simulink model "mixer_old"  (R2024b)
settings: Solver=FixedStepAuto  StartTime=0.0  StopTime=10.0  RelTol=1e-3
undefined symbols (not defined in the file or in its folder): MC_AIRMODE, MOT_SLEW_MAX, THR_MDL_FAC
libraries: simulink x58
(part 2 of 3)

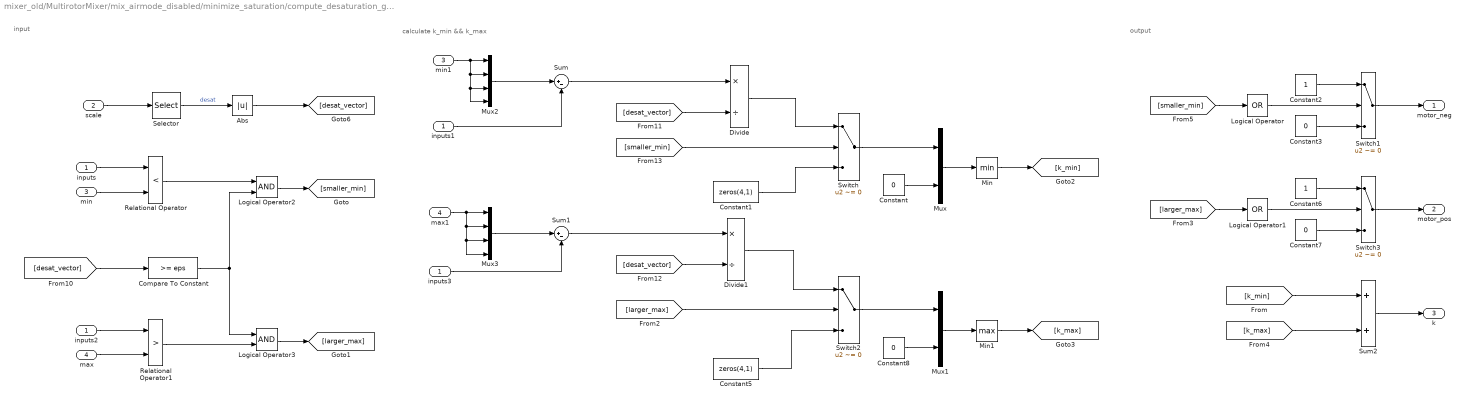
== system mixer_old/MultirotorMixer/mix_airmode_disabled/minimize_saturation/compute_desaturation_gain ==
  note: input
  note: output
  note: calculate k_min && k_max
  inputs : Inport
  scale : Inport  Port=2
  min : Inport  Port=3
  max : Inport  Port=4
  Abs : Abs  SaturateOnIntegerOverflow=off
  Compare To Constant : simulink/Logic and Bit Operations/Compare To Constant  relop=>=  const=eps  OutDataTypeStr=boolean
      settings: AttributesFormatString=%<relop>%<const>
  Constant{,3,7..8} (4 alike) : Constant  Value=0  OutDataTypeStr=single
  Constant1 : Constant  Value=zeros(4,1)  OutDataTypeStr=single
  Constant2 : Constant  OutDataTypeStr=single
  Constant5 : Constant  Value=zeros(4,1)  OutDataTypeStr=single
  Constant6 : Constant  OutDataTypeStr=single
  Divide : Product  Inputs=*/
  Divide1 : Product  Inputs=*/
  Logical Operator : Logic  Operator=OR  Inputs=1  AllPortsSameDT=off  OutDataTypeStr=boolean
  Logical Operator1 : Logic  Operator=OR  Inputs=1  AllPortsSameDT=off  OutDataTypeStr=boolean
  Logical Operator2 : Logic  AllPortsSameDT=off  OutDataTypeStr=boolean
  Logical Operator3 : Logic  AllPortsSameDT=off  OutDataTypeStr=boolean
  Min : MinMax
  Min1 : MinMax  Function=max
  Mux : Mux  Inputs=2
  Mux1 : Mux  Inputs=2
  Mux2 : Mux
  Mux3 : Mux
  Relational Operator : RelationalOperator  Operator=<  OutDataTypeStr=boolean  RndMeth=Simplest  InputSameDT=off
  Relational Operator1 : RelationalOperator  Operator=>  OutDataTypeStr=boolean  RndMeth=Simplest  InputSameDT=off
  Selector : Selector  NumberOfDimensions=2  InputPortWidth=3  IndexOptions=Select all,Index vector (dialog)  Indices=[1 3],4  OutputSizes=1,1
  Sum : Sum  Inputs=|+-
  Sum1 : Sum  Inputs=|+-
  Sum2 : Sum
  Switch{,1..3} (4 alike) : Switch  Criteria=u2 ~= 0  SaturateOnIntegerOverflow=off  InputSameDT=off
  inputs1 : InportShadow
  inputs2 : InportShadow
  inputs3 : InportShadow
  max1 : InportShadow  Port=4
  min1 : InportShadow  Port=3
  motor_neg : Outport
  motor_pos : Outport  Port=2
  k : Outport  Port=3
  wires:
  inputs/1 -> Relational Operator/1
  Mux2/1 -> Sum/1
  inputs1/1 -> Sum/2
  Sum/1 -> Divide/1
  [desat_vector] -> Divide/2
  Divide/1 -> Switch/1
  Constant1/1 -> Switch/3
  Logical Operator/1 -> Switch1/2
  Constant2/1 -> Switch1/1
  Constant3/1 -> Switch1/3
  Switch1/1 -> motor_neg/1
  inputs2/1 -> Relational Operator1/1
  [larger_max] -> Switch2/2
  Mux3/1 -> Sum1/1
  inputs3/1 -> Sum1/2
  [desat_vector] -> Divide1/2
  Sum1/1 -> Divide1/1
  Divide1/1 -> Switch2/1
  Constant5/1 -> Switch2/3
  Constant7/1 -> Switch3/3
  Constant6/1 -> Switch3/1
  Logical Operator1/1 -> Switch3/2
  Switch3/1 -> motor_pos/1
  Relational Operator/1 -> Logical Operator2/1
  [smaller_min] -> Logical Operator/1
  Relational Operator1/1 -> Logical Operator3/2
  [larger_max] -> Logical Operator1/1
  Sum2/1 -> k/1
  Compare To Constant/1 -> Logical Operator2/2, Logical Operator3/1
  Logical Operator2/1 -> [smaller_min]
  Logical Operator3/1 -> [larger_max]
  min/1 -> Relational Operator/2
  max/1 -> Relational Operator1/2
  min1/1 -> Mux2/4, Mux2/3, Mux2/2, Mux2/1
  max1/1 -> Mux3/2, Mux3/3, Mux3/4, Mux3/1
  scale/1 -> Selector/1
  Selector/1 -> Abs/1  "desat"
  Abs/1 -> [desat_vector]
  [desat_vector] -> Compare To Constant/1
  [smaller_min] -> Switch/2
  Min/1 -> [k_min]
  Min1/1 -> [k_max]
  Switch/1 -> Mux/1
  Constant/1 -> Mux/2
  Mux/1 -> Min/1
  Mux1/1 -> Min1/1
  Constant8/1 -> Mux1/2
  Switch2/1 -> Mux1/1
  [k_min] -> Sum2/1
  [k_max] -> Sum2/2

== system mixer_old/MultirotorMixer/mix_airmode_disabled/minimize_saturation1/If Action Subsystem ==
  motor_neg : Inport
  motor_pos : Inport  Port=2
  outputs : Inport  Port=3
  Action Port : ActionPort  ActionPortLabel=if(u1)
  Bus Creator : BusCreator  Inputs=3
  out : Outport
  wires:
  Bus Creator/1 -> out/1
  outputs/1 -> Bus Creator/3  "outputs"
  motor_neg/1 -> Bus Creator/1  "motor_neg"
  motor_pos/1 -> Bus Creator/2  "motor_pos"

== system mixer_old/MultirotorMixer/mix_airmode_disabled/minimize_saturation1/Subsystem ==
  k1 : Inport
  scale : Inport  Port=2
  inputs : Inport  Port=3
  Action Port : ActionPort  ActionPortLabel=else
  Bus Creator1 : BusCreator  Inputs=3
  Constant1 : Constant  Value=0  OutDataTypeStr=single
  Constant2 : Constant  OutDataTypeStr=single
  Gain : Gain  Gain=0.5
  Product : Product
  Product1 : Product
  Selector : Selector  NumberOfDimensions=2  InputPortWidth=3  IndexOptions=Select all,Index vector (dialog)  Indices=[1 3],4  OutputSizes=1,1
  Selector1 : Selector  NumberOfDimensions=2  InputPortWidth=3  IndexOptions=Select all,Index vector (dialog)  Indices=[1 3],4  OutputSizes=1,1
  Sum : Sum  Inputs=++|
  Sum1 : Sum  Inputs=|++
  compute_desaturation_gain : Subsystem
  scale1 : InportShadow  Port=2
  scale2 : InportShadow  Port=2
  out : Outport
  wires:
  Selector1/1 -> Product1/2  "desat"
  scale2/1 -> Selector1/1
  scale1/1 -> compute_desaturation_gain/2(scale)
  inputs/1 -> Sum/1
  Product/1 -> Sum/2
  Selector/1 -> Product/2  "desat"
  Constant2/1 -> compute_desaturation_gain/4(max)
  Constant1/1 -> compute_desaturation_gain/3(min)
  k1/1 -> Product/1
  Gain/1 -> Product1/1  "k2"
  Bus Creator1/1 -> out/1
  compute_desaturation_gain/1(motor_neg) -> Bus Creator1/1  "motor_neg"
  Product1/1 -> Sum1/1
  compute_desaturation_gain/3(k) -> Gain/1
  Sum1/1 -> Bus Creator1/3  "outputs"
  compute_desaturation_gain/2(motor_pos) -> Bus Creator1/2  "motor_pos"
  scale/1 -> Selector/1
  Sum/1 -> Sum1/2, compute_desaturation_gain/1(inputs)

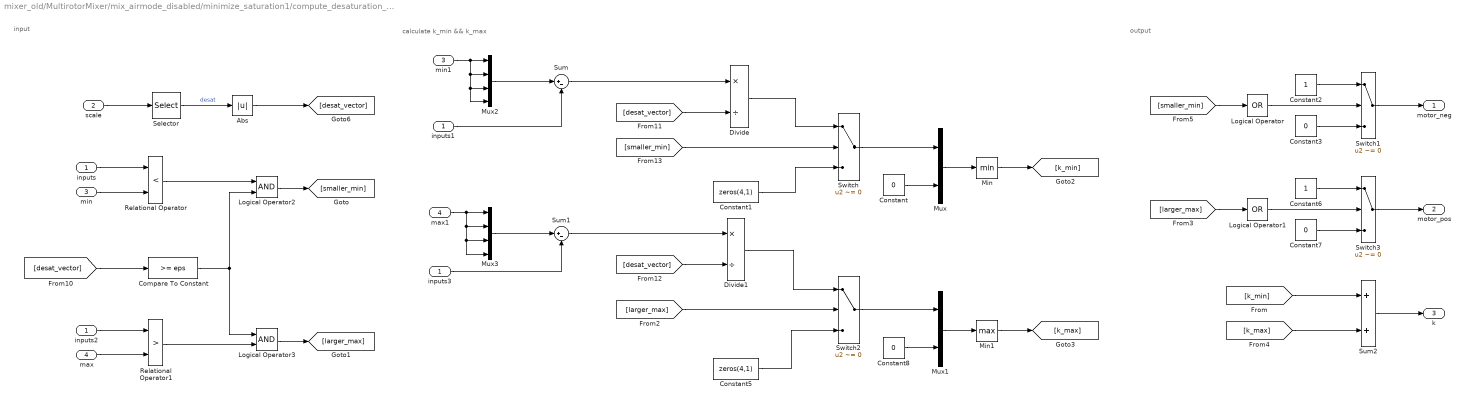
== system mixer_old/MultirotorMixer/mix_airmode_disabled/minimize_saturation1/compute_desaturation_gain ==
  note: calculate k_min && k_max
  note: output
  note: input
  inputs : Inport
  scale : Inport  Port=2
  min : Inport  Port=3
  max : Inport  Port=4
  Abs : Abs  SaturateOnIntegerOverflow=off
  Compare To Constant : simulink/Logic and Bit Operations/Compare To Constant  relop=>=  const=eps  OutDataTypeStr=boolean
      settings: AttributesFormatString=%<relop>%<const>
  Constant{,3,7..8} (4 alike) : Constant  Value=0  OutDataTypeStr=single
  Constant1 : Constant  Value=zeros(4,1)  OutDataTypeStr=single
  Constant2 : Constant  OutDataTypeStr=single
  Constant5 : Constant  Value=zeros(4,1)  OutDataTypeStr=single
  Constant6 : Constant  OutDataTypeStr=single
  Divide : Product  Inputs=*/
  Divide1 : Product  Inputs=*/
  Logical Operator : Logic  Operator=OR  Inputs=1  AllPortsSameDT=off  OutDataTypeStr=boolean
  Logical Operator1 : Logic  Operator=OR  Inputs=1  AllPortsSameDT=off  OutDataTypeStr=boolean
  Logical Operator2 : Logic  AllPortsSameDT=off  OutDataTypeStr=boolean
  Logical Operator3 : Logic  AllPortsSameDT=off  OutDataTypeStr=boolean
  Min : MinMax
  Min1 : MinMax  Function=max
  Mux : Mux  Inputs=2
  Mux1 : Mux  Inputs=2
  Mux2 : Mux
  Mux3 : Mux
  Relational Operator : RelationalOperator  Operator=<  OutDataTypeStr=boolean  RndMeth=Simplest  InputSameDT=off
  Relational Operator1 : RelationalOperator  Operator=>  OutDataTypeStr=boolean  RndMeth=Simplest  InputSameDT=off
  Selector : Selector  NumberOfDimensions=2  InputPortWidth=3  IndexOptions=Select all,Index vector (dialog)  Indices=[1 3],4  OutputSizes=1,1
  Sum : Sum  Inputs=|+-
  Sum1 : Sum  Inputs=|+-
  Sum2 : Sum
  Switch{,1..3} (4 alike) : Switch  Criteria=u2 ~= 0  SaturateOnIntegerOverflow=off  InputSameDT=off
  inputs1 : InportShadow
  inputs2 : InportShadow
  inputs3 : InportShadow
  max1 : InportShadow  Port=4
  min1 : InportShadow  Port=3
  motor_neg : Outport
  motor_pos : Outport  Port=2
  k : Outport  Port=3
  wires:
  [k_max] -> Sum2/2
  [k_min] -> Sum2/1
  Switch2/1 -> Mux1/1
  Constant8/1 -> Mux1/2
  Mux1/1 -> Min1/1
  Mux/1 -> Min/1
  Constant/1 -> Mux/2
  Switch/1 -> Mux/1
  Min1/1 -> [k_max]
  Min/1 -> [k_min]
  [smaller_min] -> Switch/2
  [desat_vector] -> Compare To Constant/1
  Abs/1 -> [desat_vector]
  Selector/1 -> Abs/1  "desat"
  scale/1 -> Selector/1
  max1/1 -> Mux3/1, Mux3/4, Mux3/3, Mux3/2
  min1/1 -> Mux2/1, Mux2/2, Mux2/3, Mux2/4
  max/1 -> Relational Operator1/2
  min/1 -> Relational Operator/2
  Logical Operator3/1 -> [larger_max]
  Logical Operator2/1 -> [smaller_min]
  Compare To Constant/1 -> Logical Operator3/1, Logical Operator2/2
  Sum2/1 -> k/1
  [larger_max] -> Logical Operator1/1
  Relational Operator1/1 -> Logical Operator3/2
  [smaller_min] -> Logical Operator/1
  Relational Operator/1 -> Logical Operator2/1
  Switch3/1 -> motor_pos/1
  Logical Operator1/1 -> Switch3/2
  Constant6/1 -> Switch3/1
  Constant7/1 -> Switch3/3
  Constant5/1 -> Switch2/3
  Divide1/1 -> Switch2/1
  Sum1/1 -> Divide1/1
  [desat_vector] -> Divide1/2
  inputs3/1 -> Sum1/2
  Mux3/1 -> Sum1/1
  [larger_max] -> Switch2/2
  inputs2/1 -> Relational Operator1/1
  Switch1/1 -> motor_neg/1
  Constant3/1 -> Switch1/3
  Constant2/1 -> Switch1/1
  Logical Operator/1 -> Switch1/2
  Constant1/1 -> Switch/3
  Divide/1 -> Switch/1
  [desat_vector] -> Divide/2
  Sum/1 -> Divide/1
  inputs1/1 -> Sum/2
  Mux2/1 -> Sum/1
  inputs/1 -> Relational Operator/1

== system mixer_old/MultirotorMixer/mix_airmode_disabled/minimize_saturation2/If Action Subsystem ==
  motor_neg : Inport
  motor_pos : Inport  Port=2
  outputs : Inport  Port=3
  Action Port : ActionPort  ActionPortLabel=if(u1)
  Bus Creator : BusCreator  Inputs=3
  out : Outport
  wires:
  motor_pos/1 -> Bus Creator/2  "motor_pos"
  motor_neg/1 -> Bus Creator/1  "motor_neg"
  outputs/1 -> Bus Creator/3  "outputs"
  Bus Creator/1 -> out/1

== system mixer_old/MultirotorMixer/mix_airmode_disabled/minimize_saturation2/Subsystem ==
  k1 : Inport
  scale : Inport  Port=2
  inputs : Inport  Port=3
  Action Port : ActionPort  ActionPortLabel=else
  Bus Creator1 : BusCreator  Inputs=3
  Constant1 : Constant  Value=0  OutDataTypeStr=single
  Constant2 : Constant  OutDataTypeStr=single
  Gain : Gain  Gain=0.5
  Product : Product
  Product1 : Product
  Selector : Selector  NumberOfDimensions=2  InputPortWidth=3  IndexOptions=Select all,Index vector (dialog)  Indices=[1 3],4  OutputSizes=1,1
  Selector1 : Selector  NumberOfDimensions=2  InputPortWidth=3  IndexOptions=Select all,Index vector (dialog)  Indices=[1 3],4  OutputSizes=1,1
  Sum : Sum  Inputs=++|
  Sum1 : Sum  Inputs=|++
  compute_desaturation_gain : Subsystem
  scale1 : InportShadow  Port=2
  scale2 : InportShadow  Port=2
  out : Outport
  wires:
  Sum/1 -> compute_desaturation_gain/1(inputs), Sum1/2
  scale/1 -> Selector/1
  compute_desaturation_gain/2(motor_pos) -> Bus Creator1/2  "motor_pos"
  Sum1/1 -> Bus Creator1/3  "outputs"
  compute_desaturation_gain/3(k) -> Gain/1
  Product1/1 -> Sum1/1
  compute_desaturation_gain/1(motor_neg) -> Bus Creator1/1  "motor_neg"
  Bus Creator1/1 -> out/1
  Gain/1 -> Product1/1  "k2"
  k1/1 -> Product/1
  Constant1/1 -> compute_desaturation_gain/3(min)
  Constant2/1 -> compute_desaturation_gain/4(max)
  Selector/1 -> Product/2  "desat"
  Product/1 -> Sum/2
  inputs/1 -> Sum/1
  scale1/1 -> compute_desaturation_gain/2(scale)
  scale2/1 -> Selector1/1
  Selector1/1 -> Product1/2  "desat"

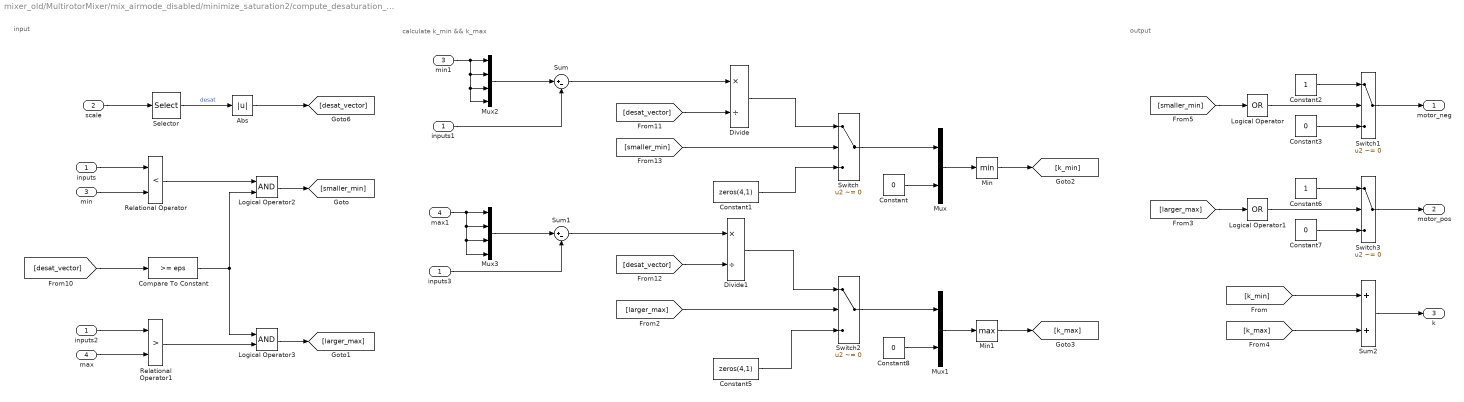
== system mixer_old/MultirotorMixer/mix_airmode_disabled/minimize_saturation2/compute_desaturation_gain ==
  note: input
  note: output
  note: calculate k_min && k_max
  inputs : Inport
  scale : Inport  Port=2
  min : Inport  Port=3
  max : Inport  Port=4
  Abs : Abs  SaturateOnIntegerOverflow=off
  Compare To Constant : simulink/Logic and Bit Operations/Compare To Constant  relop=>=  const=eps  OutDataTypeStr=boolean
      settings: AttributesFormatString=%<relop>%<const>
  Constant{,3,7..8} (4 alike) : Constant  Value=0  OutDataTypeStr=single
  Constant1 : Constant  Value=zeros(4,1)  OutDataTypeStr=single
  Constant2 : Constant  OutDataTypeStr=single
  Constant5 : Constant  Value=zeros(4,1)  OutDataTypeStr=single
  Constant6 : Constant  OutDataTypeStr=single
  Divide : Product  Inputs=*/
  Divide1 : Product  Inputs=*/
  Logical Operator : Logic  Operator=OR  Inputs=1  AllPortsSameDT=off  OutDataTypeStr=boolean
  Logical Operator1 : Logic  Operator=OR  Inputs=1  AllPortsSameDT=off  OutDataTypeStr=boolean
  Logical Operator2 : Logic  AllPortsSameDT=off  OutDataTypeStr=boolean
  Logical Operator3 : Logic  AllPortsSameDT=off  OutDataTypeStr=boolean
  Min : MinMax
  Min1 : MinMax  Function=max
  Mux : Mux  Inputs=2
  Mux1 : Mux  Inputs=2
  Mux2 : Mux
  Mux3 : Mux
  Relational Operator : RelationalOperator  Operator=<  OutDataTypeStr=boolean  RndMeth=Simplest  InputSameDT=off
  Relational Operator1 : RelationalOperator  Operator=>  OutDataTypeStr=boolean  RndMeth=Simplest  InputSameDT=off
  Selector : Selector  NumberOfDimensions=2  InputPortWidth=3  IndexOptions=Select all,Index vector (dialog)  Indices=[1 3],4  OutputSizes=1,1
  Sum : Sum  Inputs=|+-
  Sum1 : Sum  Inputs=|+-
  Sum2 : Sum
  Switch{,1..3} (4 alike) : Switch  Criteria=u2 ~= 0  SaturateOnIntegerOverflow=off  InputSameDT=off
  inputs1 : InportShadow
  inputs2 : InportShadow
  inputs3 : InportShadow
  max1 : InportShadow  Port=4
  min1 : InportShadow  Port=3
  motor_neg : Outport
  motor_pos : Outport  Port=2
  k : Outport  Port=3
  wires:
  inputs/1 -> Relational Operator/1
  Mux2/1 -> Sum/1
  inputs1/1 -> Sum/2
  Sum/1 -> Divide/1
  [desat_vector] -> Divide/2
  Divide/1 -> Switch/1
  Constant1/1 -> Switch/3
  Logical Operator/1 -> Switch1/2
  Constant2/1 -> Switch1/1
  Constant3/1 -> Switch1/3
  Switch1/1 -> motor_neg/1
  inputs2/1 -> Relational Operator1/1
  [larger_max] -> Switch2/2
  Mux3/1 -> Sum1/1
  inputs3/1 -> Sum1/2
  [desat_vector] -> Divide1/2
  Sum1/1 -> Divide1/1
  Divide1/1 -> Switch2/1
  Constant5/1 -> Switch2/3
  Constant7/1 -> Switch3/3
  Constant6/1 -> Switch3/1
  Logical Operator1/1 -> Switch3/2
  Switch3/1 -> motor_pos/1
  Relational Operator/1 -> Logical Operator2/1
  [smaller_min] -> Logical Operator/1
  Relational Operator1/1 -> Logical Operator3/2
  [larger_max] -> Logical Operator1/1
  Sum2/1 -> k/1
  Compare To Constant/1 -> Logical Operator2/2, Logical Operator3/1
  Logical Operator2/1 -> [smaller_min]
  Logical Operator3/1 -> [larger_max]
  min/1 -> Relational Operator/2
  max/1 -> Relational Operator1/2
  min1/1 -> Mux2/4, Mux2/3, Mux2/2, Mux2/1
  max1/1 -> Mux3/2, Mux3/3, Mux3/4, Mux3/1
  scale/1 -> Selector/1
  Selector/1 -> Abs/1  "desat"
  Abs/1 -> [desat_vector]
  [desat_vector] -> Compare To Constant/1
  [smaller_min] -> Switch/2
  Min/1 -> [k_min]
  Min1/1 -> [k_max]
  Switch/1 -> Mux/1
  Constant/1 -> Mux/2
  Mux/1 -> Min/1
  Mux1/1 -> Min1/1
  Constant8/1 -> Mux1/2
  Switch2/1 -> Mux1/1
  [k_min] -> Sum2/1
  [k_max] -> Sum2/2

== system mixer_old/MultirotorMixer/mix_airmode_disabled/mix_yaw/minimize_saturation2 ==
  inputs : Inport
  scale : Inport  Port=2
  min_out : Inport  Port=3
  max_out : Inport  Port=4
  reduce_only : Inport  Port=5
  Compare To Zero : simulink/Logic and Bit Operations/Compare To Zero  relop=>  OutDataTypeStr=boolean
  Data Type Conversion : DataTypeConversion  OutDataTypeStr=boolean  SaturateOnIntegerOverflow=off  RndMeth=Floor
  If : If  IfExpression=u1
  If Action Subsystem : Subsystem  TreatAsAtomicUnit=on
  Logical Operator : Logic  AllPortsSameDT=off  OutDataTypeStr=boolean
  Merge : Merge
  Subsystem : Subsystem
  compute_desaturation_gain : Subsystem
  inputs1 : InportShadow
  inputs2 : InportShadow
  scale1 : InportShadow  Port=2
  out : Outport
  wires:
  scale/1 -> compute_desaturation_gain/2(scale)
  inputs/1 -> compute_desaturation_gain/1(inputs)
  compute_desaturation_gain/3(k) -> [k1]
  reduce_only/1 -> Data Type Conversion/1
  [k1] -> Compare To Zero/1
  Data Type Conversion/1 -> Logical Operator/1
  Compare To Zero/1 -> Logical Operator/2
  Logical Operator/1 -> If/1
  Merge/1 -> out/1
  compute_desaturation_gain/2(motor_pos) -> [motor_pos]
  compute_desaturation_gain/1(motor_neg) -> [motor_neg]
  If/1 -> If Action Subsystem/Action
  scale1/1 -> Subsystem/2(scale)
  inputs2/1 -> Subsystem/3(inputs)
  If/2 -> Subsystem/Action
  [k1] -> Subsystem/1(k1)
  If Action Subsystem/1(out) -> Merge/1
  Subsystem/1(out) -> Merge/2
  [motor_pos] -> If Action Subsystem/2(motor_pos)
  [motor_neg] -> If Action Subsystem/1(motor_neg)
  inputs1/1 -> If Action Subsystem/3(outputs)
  min_out/1 -> compute_desaturation_gain/3(min)
  max_out/1 -> compute_desaturation_gain/4(max)

== system mixer_old/MultirotorMixer/mix_airmode_disabled/mix_yaw/minimize_saturation3 ==
  inputs : Inport
  scale : Inport  Port=2
  min_out : Inport  Port=3
  max_out : Inport  Port=4
  reduce_only : Inport  Port=5
  Compare To Zero : simulink/Logic and Bit Operations/Compare To Zero  relop=>  OutDataTypeStr=boolean
  Data Type Conversion : DataTypeConversion  OutDataTypeStr=boolean  SaturateOnIntegerOverflow=off  RndMeth=Floor
  If : If  IfExpression=u1
  If Action Subsystem : Subsystem  TreatAsAtomicUnit=on
  Logical Operator : Logic  AllPortsSameDT=off  OutDataTypeStr=boolean
  Merge : Merge
  Subsystem : Subsystem
  compute_desaturation_gain : Subsystem
  inputs1 : InportShadow
  inputs2 : InportShadow
  scale1 : InportShadow  Port=2
  out : Outport
  wires:
  scale/1 -> compute_desaturation_gain/2(scale)
  inputs/1 -> compute_desaturation_gain/1(inputs)
  compute_desaturation_gain/3(k) -> [k1]
  reduce_only/1 -> Data Type Conversion/1
  [k1] -> Compare To Zero/1
  Data Type Conversion/1 -> Logical Operator/1
  Compare To Zero/1 -> Logical Operator/2
  Logical Operator/1 -> If/1
  Merge/1 -> out/1
  compute_desaturation_gain/2(motor_pos) -> [motor_pos]
  compute_desaturation_gain/1(motor_neg) -> [motor_neg]
  If/1 -> If Action Subsystem/Action
  scale1/1 -> Subsystem/2(scale)
  inputs2/1 -> Subsystem/3(inputs)
  If/2 -> Subsystem/Action
  [k1] -> Subsystem/1(k1)
  If Action Subsystem/1(out) -> Merge/1
  Subsystem/1(out) -> Merge/2
  [motor_pos] -> If Action Subsystem/2(motor_pos)
  [motor_neg] -> If Action Subsystem/1(motor_neg)
  inputs1/1 -> If Action Subsystem/3(outputs)
  min_out/1 -> compute_desaturation_gain/3(min)
  max_out/1 -> compute_desaturation_gain/4(max)

== system mixer_old/MultirotorMixer/mix_airmode_rp/minimize_saturation/If Action Subsystem ==
  motor_neg : Inport
  motor_pos : Inport  Port=2
  outputs : Inport  Port=3
  Action Port : ActionPort  ActionPortLabel=if(u1)
  Bus Creator : BusCreator  Inputs=3
  out : Outport
  wires:
  motor_pos/1 -> Bus Creator/2  "motor_pos"
  motor_neg/1 -> Bus Creator/1  "motor_neg"
  outputs/1 -> Bus Creator/3  "outputs"
  Bus Creator/1 -> out/1

== system mixer_old/MultirotorMixer/mix_airmode_rp/minimize_saturation/Subsystem ==
  k1 : Inport
  scale : Inport  Port=2
  inputs : Inport  Port=3
  Action Port : ActionPort  ActionPortLabel=else
  Bus Creator1 : BusCreator  Inputs=3
  Constant1 : Constant  Value=0  OutDataTypeStr=single
  Constant2 : Constant  OutDataTypeStr=single
  Gain : Gain  Gain=0.5
  Product : Product
  Product1 : Product
  Selector : Selector  NumberOfDimensions=2  InputPortWidth=3  IndexOptions=Select all,Index vector (dialog)  Indices=[1 3],4  OutputSizes=1,1
  Selector1 : Selector  NumberOfDimensions=2  InputPortWidth=3  IndexOptions=Select all,Index vector (dialog)  Indices=[1 3],4  OutputSizes=1,1
  Sum : Sum  Inputs=++|
  Sum1 : Sum  Inputs=|++
  compute_desaturation_gain : Subsystem
  scale1 : InportShadow  Port=2
  scale2 : InportShadow  Port=2
  out : Outport
  wires:
  Sum/1 -> compute_desaturation_gain/1(inputs), Sum1/2
  scale/1 -> Selector/1
  compute_desaturation_gain/2(motor_pos) -> Bus Creator1/2  "motor_pos"
  Sum1/1 -> Bus Creator1/3  "outputs"
  compute_desaturation_gain/3(k) -> Gain/1
  Product1/1 -> Sum1/1
  compute_desaturation_gain/1(motor_neg) -> Bus Creator1/1  "motor_neg"
  Bus Creator1/1 -> out/1
  Gain/1 -> Product1/1  "k2"
  k1/1 -> Product/1
  Constant1/1 -> compute_desaturation_gain/3(min)
  Constant2/1 -> compute_desaturation_gain/4(max)
  Selector/1 -> Product/2  "desat"
  Product/1 -> Sum/2
  inputs/1 -> Sum/1
  scale1/1 -> compute_desaturation_gain/2(scale)
  scale2/1 -> Selector1/1
  Selector1/1 -> Product1/2  "desat"

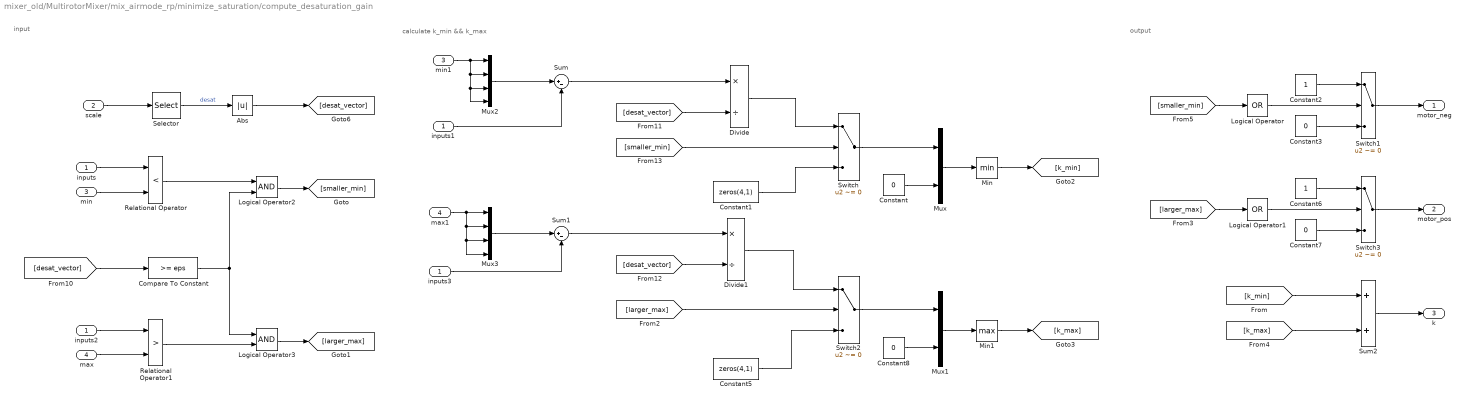
== system mixer_old/MultirotorMixer/mix_airmode_rp/minimize_saturation/compute_desaturation_gain ==
  note: input
  note: output
  note: calculate k_min && k_max
  inputs : Inport
  scale : Inport  Port=2
  min : Inport  Port=3
  max : Inport  Port=4
  Abs : Abs  SaturateOnIntegerOverflow=off
  Compare To Constant : simulink/Logic and Bit Operations/Compare To Constant  relop=>=  const=eps  OutDataTypeStr=boolean
      settings: AttributesFormatString=%<relop>%<const>
  Constant{,3,7..8} (4 alike) : Constant  Value=0  OutDataTypeStr=single
  Constant1 : Constant  Value=zeros(4,1)  OutDataTypeStr=single
  Constant2 : Constant  OutDataTypeStr=single
  Constant5 : Constant  Value=zeros(4,1)  OutDataTypeStr=single
  Constant6 : Constant  OutDataTypeStr=single
  Divide : Product  Inputs=*/
  Divide1 : Product  Inputs=*/
  Logical Operator : Logic  Operator=OR  Inputs=1  AllPortsSameDT=off  OutDataTypeStr=boolean
  Logical Operator1 : Logic  Operator=OR  Inputs=1  AllPortsSameDT=off  OutDataTypeStr=boolean
  Logical Operator2 : Logic  AllPortsSameDT=off  OutDataTypeStr=boolean
  Logical Operator3 : Logic  AllPortsSameDT=off  OutDataTypeStr=boolean
  Min : MinMax
  Min1 : MinMax  Function=max
  Mux : Mux  Inputs=2
  Mux1 : Mux  Inputs=2
  Mux2 : Mux
  Mux3 : Mux
  Relational Operator : RelationalOperator  Operator=<  OutDataTypeStr=boolean  RndMeth=Simplest  InputSameDT=off
  Relational Operator1 : RelationalOperator  Operator=>  OutDataTypeStr=boolean  RndMeth=Simplest  InputSameDT=off
  Selector : Selector  NumberOfDimensions=2  InputPortWidth=3  IndexOptions=Select all,Index vector (dialog)  Indices=[1 3],4  OutputSizes=1,1
  Sum : Sum  Inputs=|+-
  Sum1 : Sum  Inputs=|+-
  Sum2 : Sum
  Switch{,1..3} (4 alike) : Switch  Criteria=u2 ~= 0  SaturateOnIntegerOverflow=off  InputSameDT=off
  inputs1 : InportShadow
  inputs2 : InportShadow
  inputs3 : InportShadow
  max1 : InportShadow  Port=4
  min1 : InportShadow  Port=3
  motor_neg : Outport
  motor_pos : Outport  Port=2
  k : Outport  Port=3
  wires:
  inputs/1 -> Relational Operator/1
  Mux2/1 -> Sum/1
  inputs1/1 -> Sum/2
  Sum/1 -> Divide/1
  [desat_vector] -> Divide/2
  Divide/1 -> Switch/1
  Constant1/1 -> Switch/3
  Logical Operator/1 -> Switch1/2
  Constant2/1 -> Switch1/1
  Constant3/1 -> Switch1/3
  Switch1/1 -> motor_neg/1
  inputs2/1 -> Relational Operator1/1
  [larger_max] -> Switch2/2
  Mux3/1 -> Sum1/1
  inputs3/1 -> Sum1/2
  [desat_vector] -> Divide1/2
  Sum1/1 -> Divide1/1
  Divide1/1 -> Switch2/1
  Constant5/1 -> Switch2/3
  Constant7/1 -> Switch3/3
  Constant6/1 -> Switch3/1
  Logical Operator1/1 -> Switch3/2
  Switch3/1 -> motor_pos/1
  Relational Operator/1 -> Logical Operator2/1
  [smaller_min] -> Logical Operator/1
  Relational Operator1/1 -> Logical Operator3/2
  [larger_max] -> Logical Operator1/1
  Sum2/1 -> k/1
  Compare To Constant/1 -> Logical Operator2/2, Logical Operator3/1
  Logical Operator2/1 -> [smaller_min]
  Logical Operator3/1 -> [larger_max]
  min/1 -> Relational Operator/2
  max/1 -> Relational Operator1/2
  min1/1 -> Mux2/4, Mux2/3, Mux2/2, Mux2/1
  max1/1 -> Mux3/2, Mux3/3, Mux3/4, Mux3/1
  scale/1 -> Selector/1
  Selector/1 -> Abs/1  "desat"
  Abs/1 -> [desat_vector]
  [desat_vector] -> Compare To Constant/1
  [smaller_min] -> Switch/2
  Min/1 -> [k_min]
  Min1/1 -> [k_max]
  Switch/1 -> Mux/1
  Constant/1 -> Mux/2
  Mux/1 -> Min/1
  Mux1/1 -> Min1/1
  Constant8/1 -> Mux1/2
  Switch2/1 -> Mux1/1
  [k_min] -> Sum2/1
  [k_max] -> Sum2/2

== system mixer_old/MultirotorMixer/mix_airmode_rp/mix_yaw/minimize_saturation2 ==
  inputs : Inport
  scale : Inport  Port=2
  min_out : Inport  Port=3
  max_out : Inport  Port=4
  reduce_only : Inport  Port=5
  Compare To Zero : simulink/Logic and Bit Operations/Compare To Zero  relop=>  OutDataTypeStr=boolean
  Data Type Conversion : DataTypeConversion  OutDataTypeStr=boolean  SaturateOnIntegerOverflow=off  RndMeth=Floor
  If : If  IfExpression=u1
  If Action Subsystem : Subsystem  TreatAsAtomicUnit=on
  Logical Operator : Logic  AllPortsSameDT=off  OutDataTypeStr=boolean
  Merge : Merge
  Subsystem : Subsystem
  compute_desaturation_gain : Subsystem
  inputs1 : InportShadow
  inputs2 : InportShadow
  scale1 : InportShadow  Port=2
  out : Outport
  wires:
  scale/1 -> compute_desaturation_gain/2(scale)
  inputs/1 -> compute_desaturation_gain/1(inputs)
  compute_desaturation_gain/3(k) -> [k1]
  reduce_only/1 -> Data Type Conversion/1
  [k1] -> Compare To Zero/1
  Data Type Conversion/1 -> Logical Operator/1
  Compare To Zero/1 -> Logical Operator/2
  Logical Operator/1 -> If/1
  Merge/1 -> out/1
  compute_desaturation_gain/2(motor_pos) -> [motor_pos]
  compute_desaturation_gain/1(motor_neg) -> [motor_neg]
  If/1 -> If Action Subsystem/Action
  scale1/1 -> Subsystem/2(scale)
  inputs2/1 -> Subsystem/3(inputs)
  If/2 -> Subsystem/Action
  [k1] -> Subsystem/1(k1)
  If Action Subsystem/1(out) -> Merge/1
  Subsystem/1(out) -> Merge/2
  [motor_pos] -> If Action Subsystem/2(motor_pos)
  [motor_neg] -> If Action Subsystem/1(motor_neg)
  inputs1/1 -> If Action Subsystem/3(outputs)
  min_out/1 -> compute_desaturation_gain/3(min)
  max_out/1 -> compute_desaturation_gain/4(max)

== system mixer_old/MultirotorMixer/mix_airmode_rp/mix_yaw/minimize_saturation3 ==
  inputs : Inport
  scale : Inport  Port=2
  min_out : Inport  Port=3
  max_out : Inport  Port=4
  reduce_only : Inport  Port=5
  Compare To Zero : simulink/Logic and Bit Operations/Compare To Zero  relop=>  OutDataTypeStr=boolean
  Data Type Conversion : DataTypeConversion  OutDataTypeStr=boolean  SaturateOnIntegerOverflow=off  RndMeth=Floor
  If : If  IfExpression=u1
  If Action Subsystem : Subsystem  TreatAsAtomicUnit=on
  Logical Operator : Logic  AllPortsSameDT=off  OutDataTypeStr=boolean
  Merge : Merge
  Subsystem : Subsystem
  compute_desaturation_gain : Subsystem
  inputs1 : InportShadow
  inputs2 : InportShadow
  scale1 : InportShadow  Port=2
  out : Outport
  wires:
  scale/1 -> compute_desaturation_gain/2(scale)
  inputs/1 -> compute_desaturation_gain/1(inputs)
  compute_desaturation_gain/3(k) -> [k1]
  reduce_only/1 -> Data Type Conversion/1
  [k1] -> Compare To Zero/1
  Data Type Conversion/1 -> Logical Operator/1
  Compare To Zero/1 -> Logical Operator/2
  Logical Operator/1 -> If/1
  Merge/1 -> out/1
  compute_desaturation_gain/2(motor_pos) -> [motor_pos]
  compute_desaturation_gain/1(motor_neg) -> [motor_neg]
  If/1 -> If Action Subsystem/Action
  scale1/1 -> Subsystem/2(scale)
  inputs2/1 -> Subsystem/3(inputs)
  If/2 -> Subsystem/Action
  [k1] -> Subsystem/1(k1)
  If Action Subsystem/1(out) -> Merge/1
  Subsystem/1(out) -> Merge/2
  [motor_pos] -> If Action Subsystem/2(motor_pos)
  [motor_neg] -> If Action Subsystem/1(motor_neg)
  inputs1/1 -> If Action Subsystem/3(outputs)
  min_out/1 -> compute_desaturation_gain/3(min)
  max_out/1 -> compute_desaturation_gain/4(max)

== system mixer_old/MultirotorMixer/mix_airmode_rpy/minimize_saturation/If Action Subsystem ==
  motor_neg : Inport
  motor_pos : Inport  Port=2
  outputs : Inport  Port=3
  Action Port : ActionPort  ActionPortLabel=if(u1)
  Bus Creator : BusCreator  Inputs=3
  out : Outport
  wires:
  motor_pos/1 -> Bus Creator/2  "motor_pos"
  motor_neg/1 -> Bus Creator/1  "motor_neg"
  outputs/1 -> Bus Creator/3  "outputs"
  Bus Creator/1 -> out/1

== system mixer_old/MultirotorMixer/mix_airmode_rpy/minimize_saturation/Subsystem ==
  k1 : Inport
  scale : Inport  Port=2
  inputs : Inport  Port=3
  Action Port : ActionPort  ActionPortLabel=else
  Bus Creator1 : BusCreator  Inputs=3
  Constant1 : Constant  Value=0  OutDataTypeStr=single
  Constant2 : Constant  OutDataTypeStr=single
  Gain : Gain  Gain=0.5
  Product : Product
  Product1 : Product
  Selector : Selector  NumberOfDimensions=2  InputPortWidth=3  IndexOptions=Select all,Index vector (dialog)  Indices=[1 3],4  OutputSizes=1,1
  Selector1 : Selector  NumberOfDimensions=2  InputPortWidth=3  IndexOptions=Select all,Index vector (dialog)  Indices=[1 3],4  OutputSizes=1,1
  Sum : Sum  Inputs=++|
  Sum1 : Sum  Inputs=|++
  compute_desaturation_gain : Subsystem
  scale1 : InportShadow  Port=2
  scale2 : InportShadow  Port=2
  out : Outport
  wires:
  Sum/1 -> compute_desaturation_gain/1(inputs), Sum1/2
  scale/1 -> Selector/1
  compute_desaturation_gain/2(motor_pos) -> Bus Creator1/2  "motor_pos"
  Sum1/1 -> Bus Creator1/3  "outputs"
  compute_desaturation_gain/3(k) -> Gain/1
  Product1/1 -> Sum1/1
  compute_desaturation_gain/1(motor_neg) -> Bus Creator1/1  "motor_neg"
  Bus Creator1/1 -> out/1
  Gain/1 -> Product1/1  "k2"
  k1/1 -> Product/1
  Constant1/1 -> compute_desaturation_gain/3(min)
  Constant2/1 -> compute_desaturation_gain/4(max)
  Selector/1 -> Product/2  "desat"
  Product/1 -> Sum/2
  inputs/1 -> Sum/1
  scale1/1 -> compute_desaturation_gain/2(scale)
  scale2/1 -> Selector1/1
  Selector1/1 -> Product1/2  "desat"

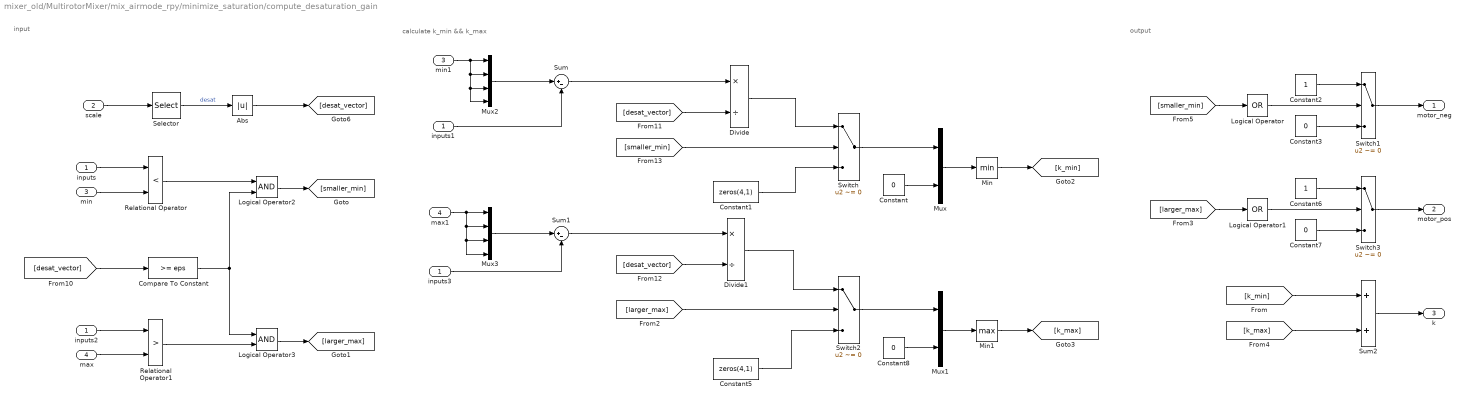
== system mixer_old/MultirotorMixer/mix_airmode_rpy/minimize_saturation/compute_desaturation_gain ==
  note: input
  note: output
  note: calculate k_min && k_max
  inputs : Inport
  scale : Inport  Port=2
  min : Inport  Port=3
  max : Inport  Port=4
  Abs : Abs  SaturateOnIntegerOverflow=off
  Compare To Constant : simulink/Logic and Bit Operations/Compare To Constant  relop=>=  const=eps  OutDataTypeStr=boolean
      settings: AttributesFormatString=%<relop>%<const>
  Constant{,3,7..8} (4 alike) : Constant  Value=0  OutDataTypeStr=single
  Constant1 : Constant  Value=zeros(4,1)  OutDataTypeStr=single
  Constant2 : Constant  OutDataTypeStr=single
  Constant5 : Constant  Value=zeros(4,1)  OutDataTypeStr=single
  Constant6 : Constant  OutDataTypeStr=single
  Divide : Product  Inputs=*/
  Divide1 : Product  Inputs=*/
  Logical Operator : Logic  Operator=OR  Inputs=1  AllPortsSameDT=off  OutDataTypeStr=boolean
  Logical Operator1 : Logic  Operator=OR  Inputs=1  AllPortsSameDT=off  OutDataTypeStr=boolean
  Logical Operator2 : Logic  AllPortsSameDT=off  OutDataTypeStr=boolean
  Logical Operator3 : Logic  AllPortsSameDT=off  OutDataTypeStr=boolean
  Min : MinMax
  Min1 : MinMax  Function=max
  Mux : Mux  Inputs=2
  Mux1 : Mux  Inputs=2
  Mux2 : Mux
  Mux3 : Mux
  Relational Operator : RelationalOperator  Operator=<  OutDataTypeStr=boolean  RndMeth=Simplest  InputSameDT=off
  Relational Operator1 : RelationalOperator  Operator=>  OutDataTypeStr=boolean  RndMeth=Simplest  InputSameDT=off
  Selector : Selector  NumberOfDimensions=2  InputPortWidth=3  IndexOptions=Select all,Index vector (dialog)  Indices=[1 3],4  OutputSizes=1,1
  Sum : Sum  Inputs=|+-
  Sum1 : Sum  Inputs=|+-
  Sum2 : Sum
  Switch{,1..3} (4 alike) : Switch  Criteria=u2 ~= 0  SaturateOnIntegerOverflow=off  InputSameDT=off
  inputs1 : InportShadow
  inputs2 : InportShadow
  inputs3 : InportShadow
  max1 : InportShadow  Port=4
  min1 : InportShadow  Port=3
  motor_neg : Outport
  motor_pos : Outport  Port=2
  k : Outport  Port=3
  wires:
  inputs/1 -> Relational Operator/1
  Mux2/1 -> Sum/1
  inputs1/1 -> Sum/2
  Sum/1 -> Divide/1
  [desat_vector] -> Divide/2
  Divide/1 -> Switch/1
  Constant1/1 -> Switch/3
  Logical Operator/1 -> Switch1/2
  Constant2/1 -> Switch1/1
  Constant3/1 -> Switch1/3
  Switch1/1 -> motor_neg/1
  inputs2/1 -> Relational Operator1/1
  [larger_max] -> Switch2/2
  Mux3/1 -> Sum1/1
  inputs3/1 -> Sum1/2
  [desat_vector] -> Divide1/2
  Sum1/1 -> Divide1/1
  Divide1/1 -> Switch2/1
  Constant5/1 -> Switch2/3
  Constant7/1 -> Switch3/3
  Constant6/1 -> Switch3/1
  Logical Operator1/1 -> Switch3/2
  Switch3/1 -> motor_pos/1
  Relational Operator/1 -> Logical Operator2/1
  [smaller_min] -> Logical Operator/1
  Relational Operator1/1 -> Logical Operator3/2
  [larger_max] -> Logical Operator1/1
  Sum2/1 -> k/1
  Compare To Constant/1 -> Logical Operator2/2, Logical Operator3/1
  Logical Operator2/1 -> [smaller_min]
  Logical Operator3/1 -> [larger_max]
  min/1 -> Relational Operator/2
  max/1 -> Relational Operator1/2
  min1/1 -> Mux2/4, Mux2/3, Mux2/2, Mux2/1
  max1/1 -> Mux3/2, Mux3/3, Mux3/4, Mux3/1
  scale/1 -> Selector/1
  Selector/1 -> Abs/1  "desat"
  Abs/1 -> [desat_vector]
  [desat_vector] -> Compare To Constant/1
  [smaller_min] -> Switch/2
  Min/1 -> [k_min]
  Min1/1 -> [k_max]
  Switch/1 -> Mux/1
  Constant/1 -> Mux/2
  Mux/1 -> Min/1
  Mux1/1 -> Min1/1
  Constant8/1 -> Mux1/2
  Switch2/1 -> Mux1/1
  [k_min] -> Sum2/1
  [k_max] -> Sum2/2

== system mixer_old/MultirotorMixer/mix_airmode_rpy/minimize_saturation1/If Action Subsystem ==
  motor_neg : Inport
  motor_pos : Inport  Port=2
  outputs : Inport  Port=3
  Action Port : ActionPort  ActionPortLabel=if(u1)
  Bus Creator : BusCreator  Inputs=3
  out : Outport
  wires:
  Bus Creator/1 -> out/1
  outputs/1 -> Bus Creator/3  "outputs"
  motor_neg/1 -> Bus Creator/1  "motor_neg"
  motor_pos/1 -> Bus Creator/2  "motor_pos"

== system mixer_old/MultirotorMixer/mix_airmode_rpy/minimize_saturation1/Subsystem ==
  k1 : Inport
  scale : Inport  Port=2
  inputs : Inport  Port=3
  Action Port : ActionPort  ActionPortLabel=else
  Bus Creator1 : BusCreator  Inputs=3
  Constant1 : Constant  Value=0  OutDataTypeStr=single
  Constant2 : Constant  OutDataTypeStr=single
  Gain : Gain  Gain=0.5
  Product : Product
  Product1 : Product
  Selector : Selector  NumberOfDimensions=2  InputPortWidth=3  IndexOptions=Select all,Index vector (dialog)  Indices=[1 3],4  OutputSizes=1,1
  Selector1 : Selector  NumberOfDimensions=2  InputPortWidth=3  IndexOptions=Select all,Index vector (dialog)  Indices=[1 3],4  OutputSizes=1,1
  Sum : Sum  Inputs=++|
  Sum1 : Sum  Inputs=|++
  compute_desaturation_gain : Subsystem
  scale1 : InportShadow  Port=2
  scale2 : InportShadow  Port=2
  out : Outport
  wires:
  Selector1/1 -> Product1/2  "desat"
  scale2/1 -> Selector1/1
  scale1/1 -> compute_desaturation_gain/2(scale)
  inputs/1 -> Sum/1
  Product/1 -> Sum/2
  Selector/1 -> Product/2  "desat"
  Constant2/1 -> compute_desaturation_gain/4(max)
  Constant1/1 -> compute_desaturation_gain/3(min)
  k1/1 -> Product/1
  Gain/1 -> Product1/1  "k2"
  Bus Creator1/1 -> out/1
  compute_desaturation_gain/1(motor_neg) -> Bus Creator1/1  "motor_neg"
  Product1/1 -> Sum1/1
  compute_desaturation_gain/3(k) -> Gain/1
  Sum1/1 -> Bus Creator1/3  "outputs"
  compute_desaturation_gain/2(motor_pos) -> Bus Creator1/2  "motor_pos"
  scale/1 -> Selector/1
  Sum/1 -> Sum1/2, compute_desaturation_gain/1(inputs)

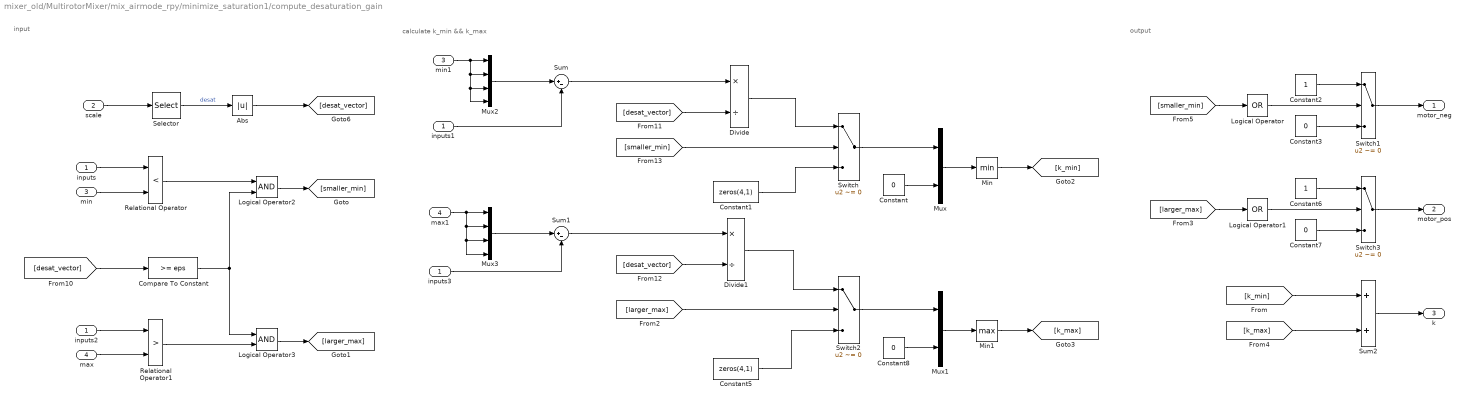
== system mixer_old/MultirotorMixer/mix_airmode_rpy/minimize_saturation1/compute_desaturation_gain ==
  note: calculate k_min && k_max
  note: output
  note: input
  inputs : Inport
  scale : Inport  Port=2
  min : Inport  Port=3
  max : Inport  Port=4
  Abs : Abs  SaturateOnIntegerOverflow=off
  Compare To Constant : simulink/Logic and Bit Operations/Compare To Constant  relop=>=  const=eps  OutDataTypeStr=boolean
      settings: AttributesFormatString=%<relop>%<const>
  Constant{,3,7..8} (4 alike) : Constant  Value=0  OutDataTypeStr=single
  Constant1 : Constant  Value=zeros(4,1)  OutDataTypeStr=single
  Constant2 : Constant  OutDataTypeStr=single
  Constant5 : Constant  Value=zeros(4,1)  OutDataTypeStr=single
  Constant6 : Constant  OutDataTypeStr=single
  Divide : Product  Inputs=*/
  Divide1 : Product  Inputs=*/
  Logical Operator : Logic  Operator=OR  Inputs=1  AllPortsSameDT=off  OutDataTypeStr=boolean
  Logical Operator1 : Logic  Operator=OR  Inputs=1  AllPortsSameDT=off  OutDataTypeStr=boolean
  Logical Operator2 : Logic  AllPortsSameDT=off  OutDataTypeStr=boolean
  Logical Operator3 : Logic  AllPortsSameDT=off  OutDataTypeStr=boolean
  Min : MinMax
  Min1 : MinMax  Function=max
  Mux : Mux  Inputs=2
  Mux1 : Mux  Inputs=2
  Mux2 : Mux
  Mux3 : Mux
  Relational Operator : RelationalOperator  Operator=<  OutDataTypeStr=boolean  RndMeth=Simplest  InputSameDT=off
  Relational Operator1 : RelationalOperator  Operator=>  OutDataTypeStr=boolean  RndMeth=Simplest  InputSameDT=off
  Selector : Selector  NumberOfDimensions=2  InputPortWidth=3  IndexOptions=Select all,Index vector (dialog)  Indices=[1 3],4  OutputSizes=1,1
  Sum : Sum  Inputs=|+-
  Sum1 : Sum  Inputs=|+-
  Sum2 : Sum
  Switch{,1..3} (4 alike) : Switch  Criteria=u2 ~= 0  SaturateOnIntegerOverflow=off  InputSameDT=off
  inputs1 : InportShadow
  inputs2 : InportShadow
  inputs3 : InportShadow
  max1 : InportShadow  Port=4
  min1 : InportShadow  Port=3
  motor_neg : Outport
  motor_pos : Outport  Port=2
  k : Outport  Port=3
  wires:
  [k_max] -> Sum2/2
  [k_min] -> Sum2/1
  Switch2/1 -> Mux1/1
  Constant8/1 -> Mux1/2
  Mux1/1 -> Min1/1
  Mux/1 -> Min/1
  Constant/1 -> Mux/2
  Switch/1 -> Mux/1
  Min1/1 -> [k_max]
  Min/1 -> [k_min]
  [smaller_min] -> Switch/2
  [desat_vector] -> Compare To Constant/1
  Abs/1 -> [desat_vector]
  Selector/1 -> Abs/1  "desat"
  scale/1 -> Selector/1
  max1/1 -> Mux3/1, Mux3/4, Mux3/3, Mux3/2
  min1/1 -> Mux2/1, Mux2/2, Mux2/3, Mux2/4
  max/1 -> Relational Operator1/2
  min/1 -> Relational Operator/2
  Logical Operator3/1 -> [larger_max]
  Logical Operator2/1 -> [smaller_min]
  Compare To Constant/1 -> Logical Operator3/1, Logical Operator2/2
  Sum2/1 -> k/1
  [larger_max] -> Logical Operator1/1
  Relational Operator1/1 -> Logical Operator3/2
  [smaller_min] -> Logical Operator/1
  Relational Operator/1 -> Logical Operator2/1
  Switch3/1 -> motor_pos/1
  Logical Operator1/1 -> Switch3/2
  Constant6/1 -> Switch3/1
  Constant7/1 -> Switch3/3
  Constant5/1 -> Switch2/3
  Divide1/1 -> Switch2/1
  Sum1/1 -> Divide1/1
  [desat_vector] -> Divide1/2
  inputs3/1 -> Sum1/2
  Mux3/1 -> Sum1/1
  [larger_max] -> Switch2/2
  inputs2/1 -> Relational Operator1/1
  Switch1/1 -> motor_neg/1
  Constant3/1 -> Switch1/3
  Constant2/1 -> Switch1/1
  Logical Operator/1 -> Switch1/2
  Constant1/1 -> Switch/3
  Divide/1 -> Switch/1
  [desat_vector] -> Divide/2
  Sum/1 -> Divide/1
  inputs1/1 -> Sum/2
  Mux2/1 -> Sum/1
  inputs/1 -> Relational Operator/1

== system mixer_old/MultirotorMixer/apply_thrust_model/slew_rate_limit/cal_delta_out_max/If Action Subsystem ==
  MOT_SLEW_MAX : Inport
  Action Port : ActionPort  ActionPortLabel=case [ 1 ]:
  Divide : Product  Inputs=*/
  Gain : Gain  Gain=2000  OutDataTypeStr=single
  PWM_DEFAULT_MAX : Constant  Value=2000  OutDataTypeStr=single
  PWM_DEFAULT_MIN : Constant  Value=1000  OutDataTypeStr=single
  Sum2 : Sum  Inputs=|+-
  Weighted Sample Time : SampleTimeMath  TsampMathOp=*
  Out1 : Outport
  wires:
  PWM_DEFAULT_MAX/1 -> Sum2/1
  PWM_DEFAULT_MIN/1 -> Sum2/2
  Sum2/1 -> Divide/1
  Weighted Sample Time/1 -> Gain/1
  Divide/1 -> Weighted Sample Time/1
  Gain/1 -> Out1/1
  MOT_SLEW_MAX/1 -> Divide/2

== system mixer_old/MultirotorMixer/apply_thrust_model/slew_rate_limit/cal_delta_out_max/If Action Subsystem1 ==
  In1 : Inport
  Action Port : ActionPort  ActionPortLabel=default:
  Out1 : Outport
  wires:
  In1/1 -> Out1/1

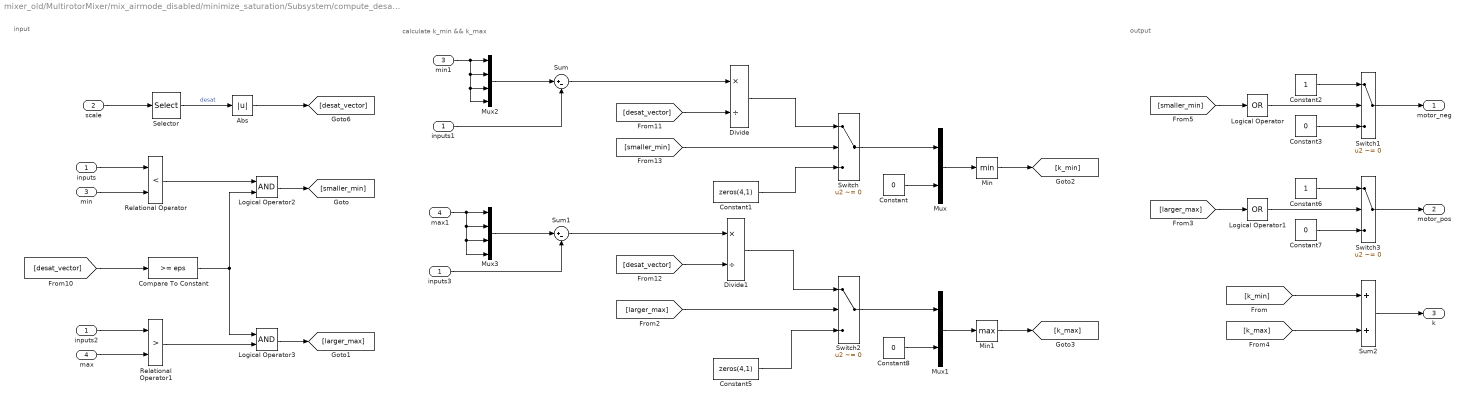
== system mixer_old/MultirotorMixer/mix_airmode_disabled/minimize_saturation/Subsystem/compute_desaturation_gain ==
  note: input
  note: output
  note: calculate k_min && k_max
  inputs : Inport
  scale : Inport  Port=2
  min : Inport  Port=3
  max : Inport  Port=4
  Abs : Abs  SaturateOnIntegerOverflow=off
  Compare To Constant : simulink/Logic and Bit Operations/Compare To Constant  relop=>=  const=eps  OutDataTypeStr=boolean
      settings: AttributesFormatString=%<relop>%<const>
  Constant{,3,7..8} (4 alike) : Constant  Value=0  OutDataTypeStr=single
  Constant1 : Constant  Value=zeros(4,1)  OutDataTypeStr=single
  Constant2 : Constant  OutDataTypeStr=single
  Constant5 : Constant  Value=zeros(4,1)  OutDataTypeStr=single
  Constant6 : Constant  OutDataTypeStr=single
  Divide : Product  Inputs=*/
  Divide1 : Product  Inputs=*/
  Logical Operator : Logic  Operator=OR  Inputs=1  AllPortsSameDT=off  OutDataTypeStr=boolean
  Logical Operator1 : Logic  Operator=OR  Inputs=1  AllPortsSameDT=off  OutDataTypeStr=boolean
  Logical Operator2 : Logic  AllPortsSameDT=off  OutDataTypeStr=boolean
  Logical Operator3 : Logic  AllPortsSameDT=off  OutDataTypeStr=boolean
  Min : MinMax
  Min1 : MinMax  Function=max
  Mux : Mux  Inputs=2
  Mux1 : Mux  Inputs=2
  Mux2 : Mux
  Mux3 : Mux
  Relational Operator : RelationalOperator  Operator=<  OutDataTypeStr=boolean  RndMeth=Simplest  InputSameDT=off
  Relational Operator1 : RelationalOperator  Operator=>  OutDataTypeStr=boolean  RndMeth=Simplest  InputSameDT=off
  Selector : Selector  NumberOfDimensions=2  InputPortWidth=3  IndexOptions=Select all,Index vector (dialog)  Indices=[1 3],4  OutputSizes=1,1
  Sum : Sum  Inputs=|+-
  Sum1 : Sum  Inputs=|+-
  Sum2 : Sum
  Switch{,1..3} (4 alike) : Switch  Criteria=u2 ~= 0  SaturateOnIntegerOverflow=off  InputSameDT=off
  inputs1 : InportShadow
  inputs2 : InportShadow
  inputs3 : InportShadow
  max1 : InportShadow  Port=4
  min1 : InportShadow  Port=3
  motor_neg : Outport
  motor_pos : Outport  Port=2
  k : Outport  Port=3
  wires:
  inputs/1 -> Relational Operator/1
  Mux2/1 -> Sum/1
  inputs1/1 -> Sum/2
  Sum/1 -> Divide/1
  [desat_vector] -> Divide/2
  Divide/1 -> Switch/1
  Constant1/1 -> Switch/3
  Logical Operator/1 -> Switch1/2
  Constant2/1 -> Switch1/1
  Constant3/1 -> Switch1/3
  Switch1/1 -> motor_neg/1
  inputs2/1 -> Relational Operator1/1
  [larger_max] -> Switch2/2
  Mux3/1 -> Sum1/1
  inputs3/1 -> Sum1/2
  [desat_vector] -> Divide1/2
  Sum1/1 -> Divide1/1
  Divide1/1 -> Switch2/1
  Constant5/1 -> Switch2/3
  Constant7/1 -> Switch3/3
  Constant6/1 -> Switch3/1
  Logical Operator1/1 -> Switch3/2
  Switch3/1 -> motor_pos/1
  Relational Operator/1 -> Logical Operator2/1
  [smaller_min] -> Logical Operator/1
  Relational Operator1/1 -> Logical Operator3/2
  [larger_max] -> Logical Operator1/1
  Sum2/1 -> k/1
  Compare To Constant/1 -> Logical Operator2/2, Logical Operator3/1
  Logical Operator2/1 -> [smaller_min]
  Logical Operator3/1 -> [larger_max]
  min/1 -> Relational Operator/2
  max/1 -> Relational Operator1/2
  min1/1 -> Mux2/4, Mux2/3, Mux2/2, Mux2/1
  max1/1 -> Mux3/2, Mux3/3, Mux3/4, Mux3/1
  scale/1 -> Selector/1
  Selector/1 -> Abs/1  "desat"
  Abs/1 -> [desat_vector]
  [desat_vector] -> Compare To Constant/1
  [smaller_min] -> Switch/2
  Min/1 -> [k_min]
  Min1/1 -> [k_max]
  Switch/1 -> Mux/1
  Constant/1 -> Mux/2
  Mux/1 -> Min/1
  Mux1/1 -> Min1/1
  Constant8/1 -> Mux1/2
  Switch2/1 -> Mux1/1
  [k_min] -> Sum2/1
  [k_max] -> Sum2/2

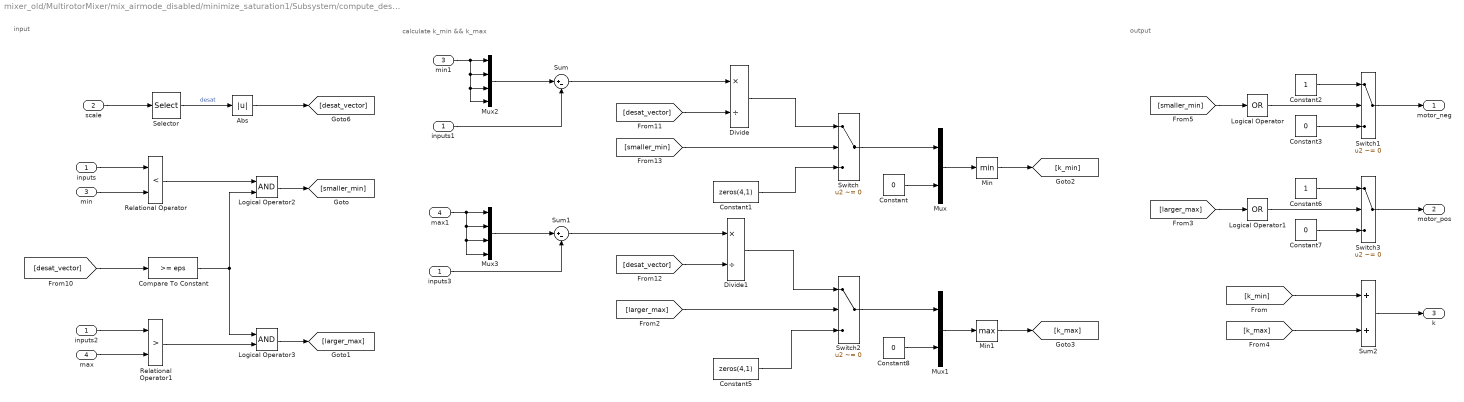
== system mixer_old/MultirotorMixer/mix_airmode_disabled/minimize_saturation1/Subsystem/compute_desaturation_gain ==
  note: calculate k_min && k_max
  note: output
  note: input
  inputs : Inport
  scale : Inport  Port=2
  min : Inport  Port=3
  max : Inport  Port=4
  Abs : Abs  SaturateOnIntegerOverflow=off
  Compare To Constant : simulink/Logic and Bit Operations/Compare To Constant  relop=>=  const=eps  OutDataTypeStr=boolean
      settings: AttributesFormatString=%<relop>%<const>
  Constant{,3,7..8} (4 alike) : Constant  Value=0  OutDataTypeStr=single
  Constant1 : Constant  Value=zeros(4,1)  OutDataTypeStr=single
  Constant2 : Constant  OutDataTypeStr=single
  Constant5 : Constant  Value=zeros(4,1)  OutDataTypeStr=single
  Constant6 : Constant  OutDataTypeStr=single
  Divide : Product  Inputs=*/
  Divide1 : Product  Inputs=*/
  Logical Operator : Logic  Operator=OR  Inputs=1  AllPortsSameDT=off  OutDataTypeStr=boolean
  Logical Operator1 : Logic  Operator=OR  Inputs=1  AllPortsSameDT=off  OutDataTypeStr=boolean
  Logical Operator2 : Logic  AllPortsSameDT=off  OutDataTypeStr=boolean
  Logical Operator3 : Logic  AllPortsSameDT=off  OutDataTypeStr=boolean
  Min : MinMax
  Min1 : MinMax  Function=max
  Mux : Mux  Inputs=2
  Mux1 : Mux  Inputs=2
  Mux2 : Mux
  Mux3 : Mux
  Relational Operator : RelationalOperator  Operator=<  OutDataTypeStr=boolean  RndMeth=Simplest  InputSameDT=off
  Relational Operator1 : RelationalOperator  Operator=>  OutDataTypeStr=boolean  RndMeth=Simplest  InputSameDT=off
  Selector : Selector  NumberOfDimensions=2  InputPortWidth=3  IndexOptions=Select all,Index vector (dialog)  Indices=[1 3],4  OutputSizes=1,1
  Sum : Sum  Inputs=|+-
  Sum1 : Sum  Inputs=|+-
  Sum2 : Sum
  Switch{,1..3} (4 alike) : Switch  Criteria=u2 ~= 0  SaturateOnIntegerOverflow=off  InputSameDT=off
  inputs1 : InportShadow
  inputs2 : InportShadow
  inputs3 : InportShadow
  max1 : InportShadow  Port=4
  min1 : InportShadow  Port=3
  motor_neg : Outport
  motor_pos : Outport  Port=2
  k : Outport  Port=3
  wires:
  [k_max] -> Sum2/2
  [k_min] -> Sum2/1
  Switch2/1 -> Mux1/1
  Constant8/1 -> Mux1/2
  Mux1/1 -> Min1/1
  Mux/1 -> Min/1
  Constant/1 -> Mux/2
  Switch/1 -> Mux/1
  Min1/1 -> [k_max]
  Min/1 -> [k_min]
  [smaller_min] -> Switch/2
  [desat_vector] -> Compare To Constant/1
  Abs/1 -> [desat_vector]
  Selector/1 -> Abs/1  "desat"
  scale/1 -> Selector/1
  max1/1 -> Mux3/1, Mux3/4, Mux3/3, Mux3/2
  min1/1 -> Mux2/1, Mux2/2, Mux2/3, Mux2/4
  max/1 -> Relational Operator1/2
  min/1 -> Relational Operator/2
  Logical Operator3/1 -> [larger_max]
  Logical Operator2/1 -> [smaller_min]
  Compare To Constant/1 -> Logical Operator3/1, Logical Operator2/2
  Sum2/1 -> k/1
  [larger_max] -> Logical Operator1/1
  Relational Operator1/1 -> Logical Operator3/2
  [smaller_min] -> Logical Operator/1
  Relational Operator/1 -> Logical Operator2/1
  Switch3/1 -> motor_pos/1
  Logical Operator1/1 -> Switch3/2
  Constant6/1 -> Switch3/1
  Constant7/1 -> Switch3/3
  Constant5/1 -> Switch2/3
  Divide1/1 -> Switch2/1
  Sum1/1 -> Divide1/1
  [desat_vector] -> Divide1/2
  inputs3/1 -> Sum1/2
  Mux3/1 -> Sum1/1
  [larger_max] -> Switch2/2
  inputs2/1 -> Relational Operator1/1
  Switch1/1 -> motor_neg/1
  Constant3/1 -> Switch1/3
  Constant2/1 -> Switch1/1
  Logical Operator/1 -> Switch1/2
  Constant1/1 -> Switch/3
  Divide/1 -> Switch/1
  [desat_vector] -> Divide/2
  Sum/1 -> Divide/1
  inputs1/1 -> Sum/2
  Mux2/1 -> Sum/1
  inputs/1 -> Relational Operator/1

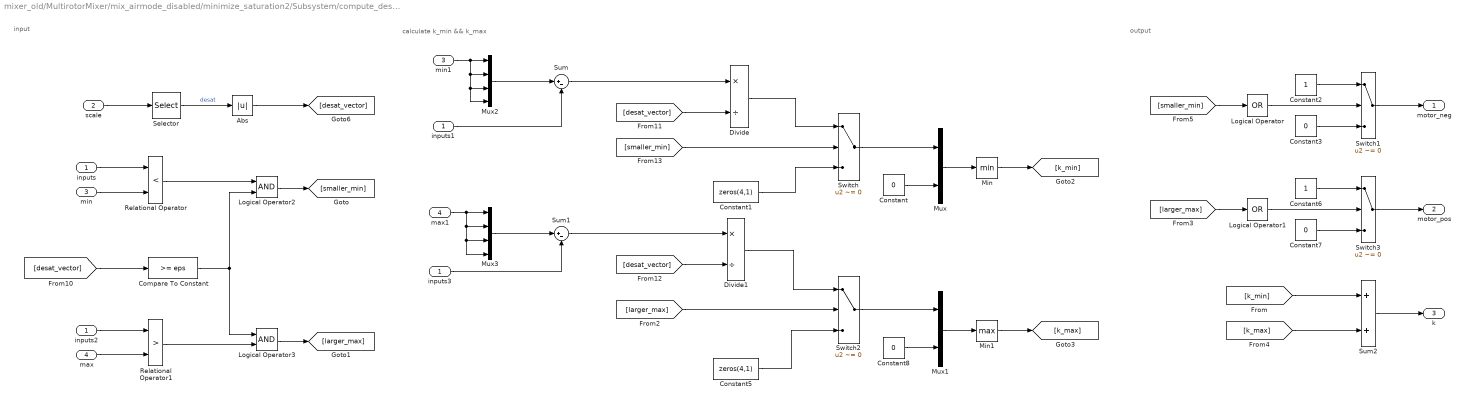
== system mixer_old/MultirotorMixer/mix_airmode_disabled/minimize_saturation2/Subsystem/compute_desaturation_gain ==
  note: input
  note: output
  note: calculate k_min && k_max
  inputs : Inport
  scale : Inport  Port=2
  min : Inport  Port=3
  max : Inport  Port=4
  Abs : Abs  SaturateOnIntegerOverflow=off
  Compare To Constant : simulink/Logic and Bit Operations/Compare To Constant  relop=>=  const=eps  OutDataTypeStr=boolean
      settings: AttributesFormatString=%<relop>%<const>
  Constant{,3,7..8} (4 alike) : Constant  Value=0  OutDataTypeStr=single
  Constant1 : Constant  Value=zeros(4,1)  OutDataTypeStr=single
  Constant2 : Constant  OutDataTypeStr=single
  Constant5 : Constant  Value=zeros(4,1)  OutDataTypeStr=single
  Constant6 : Constant  OutDataTypeStr=single
  Divide : Product  Inputs=*/
  Divide1 : Product  Inputs=*/
  Logical Operator : Logic  Operator=OR  Inputs=1  AllPortsSameDT=off  OutDataTypeStr=boolean
  Logical Operator1 : Logic  Operator=OR  Inputs=1  AllPortsSameDT=off  OutDataTypeStr=boolean
  Logical Operator2 : Logic  AllPortsSameDT=off  OutDataTypeStr=boolean
  Logical Operator3 : Logic  AllPortsSameDT=off  OutDataTypeStr=boolean
  Min : MinMax
  Min1 : MinMax  Function=max
  Mux : Mux  Inputs=2
  Mux1 : Mux  Inputs=2
  Mux2 : Mux
  Mux3 : Mux
  Relational Operator : RelationalOperator  Operator=<  OutDataTypeStr=boolean  RndMeth=Simplest  InputSameDT=off
  Relational Operator1 : RelationalOperator  Operator=>  OutDataTypeStr=boolean  RndMeth=Simplest  InputSameDT=off
  Selector : Selector  NumberOfDimensions=2  InputPortWidth=3  IndexOptions=Select all,Index vector (dialog)  Indices=[1 3],4  OutputSizes=1,1
  Sum : Sum  Inputs=|+-
  Sum1 : Sum  Inputs=|+-
  Sum2 : Sum
  Switch{,1..3} (4 alike) : Switch  Criteria=u2 ~= 0  SaturateOnIntegerOverflow=off  InputSameDT=off
  inputs1 : InportShadow
  inputs2 : InportShadow
  inputs3 : InportShadow
  max1 : InportShadow  Port=4
  min1 : InportShadow  Port=3
  motor_neg : Outport
  motor_pos : Outport  Port=2
  k : Outport  Port=3
  wires:
  inputs/1 -> Relational Operator/1
  Mux2/1 -> Sum/1
  inputs1/1 -> Sum/2
  Sum/1 -> Divide/1
  [desat_vector] -> Divide/2
  Divide/1 -> Switch/1
  Constant1/1 -> Switch/3
  Logical Operator/1 -> Switch1/2
  Constant2/1 -> Switch1/1
  Constant3/1 -> Switch1/3
  Switch1/1 -> motor_neg/1
  inputs2/1 -> Relational Operator1/1
  [larger_max] -> Switch2/2
  Mux3/1 -> Sum1/1
  inputs3/1 -> Sum1/2
  [desat_vector] -> Divide1/2
  Sum1/1 -> Divide1/1
  Divide1/1 -> Switch2/1
  Constant5/1 -> Switch2/3
  Constant7/1 -> Switch3/3
  Constant6/1 -> Switch3/1
  Logical Operator1/1 -> Switch3/2
  Switch3/1 -> motor_pos/1
  Relational Operator/1 -> Logical Operator2/1
  [smaller_min] -> Logical Operator/1
  Relational Operator1/1 -> Logical Operator3/2
  [larger_max] -> Logical Operator1/1
  Sum2/1 -> k/1
  Compare To Constant/1 -> Logical Operator2/2, Logical Operator3/1
  Logical Operator2/1 -> [smaller_min]
  Logical Operator3/1 -> [larger_max]
  min/1 -> Relational Operator/2
  max/1 -> Relational Operator1/2
  min1/1 -> Mux2/4, Mux2/3, Mux2/2, Mux2/1
  max1/1 -> Mux3/2, Mux3/3, Mux3/4, Mux3/1
  scale/1 -> Selector/1
  Selector/1 -> Abs/1  "desat"
  Abs/1 -> [desat_vector]
  [desat_vector] -> Compare To Constant/1
  [smaller_min] -> Switch/2
  Min/1 -> [k_min]
  Min1/1 -> [k_max]
  Switch/1 -> Mux/1
  Constant/1 -> Mux/2
  Mux/1 -> Min/1
  Mux1/1 -> Min1/1
  Constant8/1 -> Mux1/2
  Switch2/1 -> Mux1/1
  [k_min] -> Sum2/1
  [k_max] -> Sum2/2

== system mixer_old/MultirotorMixer/mix_airmode_disabled/mix_yaw/minimize_saturation2/If Action Subsystem ==
  motor_neg : Inport
  motor_pos : Inport  Port=2
  outputs : Inport  Port=3
  Action Port : ActionPort  ActionPortLabel=if(u1)
  Bus Creator : BusCreator  Inputs=3
  out : Outport
  wires:
  motor_pos/1 -> Bus Creator/2  "motor_pos"
  motor_neg/1 -> Bus Creator/1  "motor_neg"
  outputs/1 -> Bus Creator/3  "outputs"
  Bus Creator/1 -> out/1
